simulink model "chap13_3sim"  (Simulink 8.3)
settings: Solver=ode45  StartTime=0.0  StopTime=10  RelTol=1e-5
settings Model: Creator=ljk  LastModifiedBy=Administrator  ExtModeTrigMode=oneshot  ExtModeArmWhenConnect=off
settings DataIOCC: LimitDataPoints=off  SignalLoggingName=sigsOut
settings OptimizationCC: BooleanDataType=off  ExpressionDepthLimit=2147483647  InitFltsAndDblsToZero=on
settings DebuggingCC: SaveWithParameterizedLinksMsg=none  SignalResolutionControl=TryResolveAllWithWarning  SolverPrmCheckMsg=none  MultiTaskDSMMsg=warning  MultiTaskCondExecSysMsg=none  FcnCallInpInsideContextMsg=UseLocalSettings
settings HardwareCC: TargetUnknown=on
settings RTWCC: IncludeERTFirstTime=on
settings GRTTargetCC: TargetFcnLib=ansi_tfl_tmw.mat

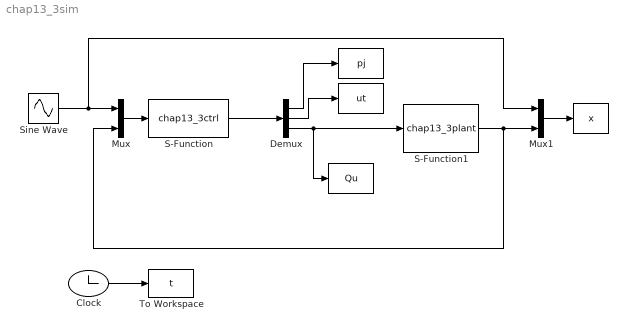
== system chap13_3sim ==
  " " : ToWorkspace  VariableName=pj  SampleTime=-1
  "  " : ToWorkspace  VariableName=x  SampleTime=-1
  "   " : ToWorkspace  VariableName=ut  SampleTime=-1
  "      " : ToWorkspace  VariableName=Qu  SampleTime=-1
  Clock : Clock
  Demux : Demux  Outputs=3
  Mux : Mux  Inputs=2
  Mux1 : Mux  Inputs=2
  S-Function : S-Function  FunctionName=chap13_3ctrl  EnableBusSupport=off
  S-Function1 : S-Function  FunctionName=chap13_3plant  EnableBusSupport=off
  Sine Wave : Sin  SampleTime=0
  To Workspace : ToWorkspace  VariableName=t  SampleTime=-1
  wires:
  S-Function1/1 -> Mux/2, Mux1/2
  Clock/1 -> To Workspace/1
  S-Function/1 -> Demux/1
  Demux/1 -> " "/1
  Mux/1 -> S-Function/1
  Sine Wave/1 -> Mux/1, Mux1/1
  Mux1/1 -> "  "/1
  Demux/3 -> S-Function1/1, "      "/1
  Demux/2 -> "   "/1
